simulink model "lab6"  (R2019b)
settings: Solver=FixedStepDiscrete  StartTime=0.0  StopTime=inf  RelTol=1e-3
values from neighbouring files (symbols this model uses):
  model_skory = createSkinModel2(RGB,BW)    [Lab6.m]
undefined symbols (not defined in the file or in its folder): gray, Rec, SDTV
libraries: visionconversions x1, visiontextngfix x1, dspvision x1
settings Model: Creator=fw2ty  LastModifiedBy=fw2ty

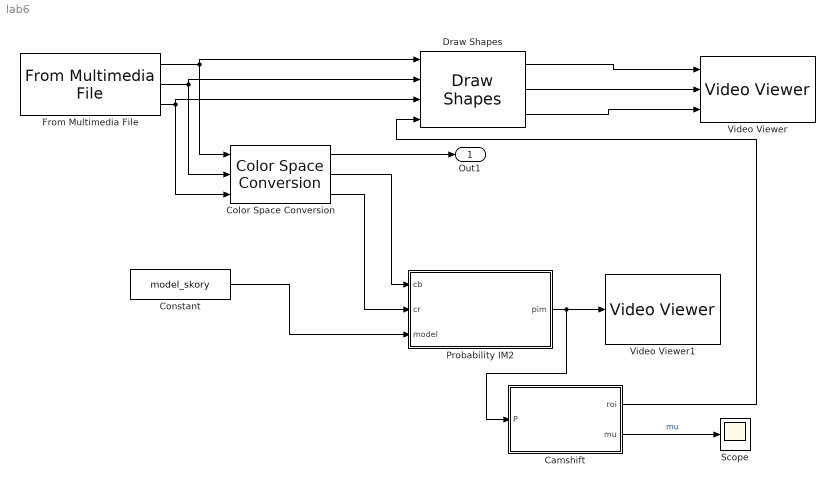
== system lab6 ==
  Camshift : MATLAB Function  TreatAsAtomicUnit=on
  Color Space Conversion : visionconversions/Color Space  Conversion  conversion=Obsolete  conversionActive=R'G'B' to Y'CbCr  wp_str=D65  rec=Rec. 601 (SDTV)  sys=1125/60/2:1  imagePorts=Separate color signals
  Constant : Constant  Value=model_skory
  Draw Shapes : visiontextngfix/Draw Shapes  shape=Rectangles  fill=off  lineWidth=1  fillClrSource=Specify via dialog  display=Black  intensity=200  color=[200 255 100]  opacity=0.6  viewport=Entire image  antialiasing=off  inType=Obsolete  imagePorts=Separate color signals  roundingMode=Floor  overflowMode=off  memoryMode=Specify word length  memoryWordLength=16  prodOutputMode=Binary point scaling  prodOutputWordLength=32  prodOutputFracLength=14  prodOutputSlope=2^-14  accumSlope=2^-14  memoryFracLength=15
      settings: SourceProductName=Computer Vision Toolbox
  From Multimedia File : dspvision/From Multimedia File  inputFilename=video.avi  readRange=[1 Inf]  loop=on  numPlays=inf  outputStreams=Video only  videoDataType=uint8  audioDataType=int16  inheritSampleTime=on  userDefinedSampleTime=1/30  noAudioOutput=off  isIntensityVideo=off  fourcc=RGB  colorVideoFormat=Separate color signals  outputEOF=off  dataOrg=Column-major  audioFrameSize=1024  computeAudioFrameSize=off  outSamplingMode=Sample based
      settings: SourceProductName=DSP System Toolbox  SourceProductBaseCode=DS
  Probability IM2 : MATLAB Function  TreatAsAtomicUnit=on
  Scope : Scope
  Video Viewer : VideoViewer  imagePorts=separate color signals  colormapValue=gray(256)  FigPos=[370 695 408 302]
  Video Viewer1 : VideoViewer  useColorMap=on  specRange=on  maxInputVal=1  FigPos=[845 857 587 499]
  Out1 : Outport
  wires:
  From Multimedia File/1 -> Draw Shapes/1, Color Space Conversion/1
  From Multimedia File/2 -> Color Space Conversion/2, Draw Shapes/2
  From Multimedia File/3 -> Color Space Conversion/3, Draw Shapes/3
  Color Space Conversion/2 -> Probability IM2/1(cb)
  Color Space Conversion/3 -> Probability IM2/2(cr)
  Constant/1 -> Probability IM2/3(model)
  Probability IM2/1(pim) -> Camshift/1(P), Video Viewer1/1
  Color Space Conversion/1 -> Out1/1
  Camshift/1(roi) -> Draw Shapes/4
  Draw Shapes/1 -> Video Viewer/1
  Draw Shapes/2 -> Video Viewer/2
  Draw Shapes/3 -> Video Viewer/3
  Camshift/2(mu) -> Scope/1  "mu"

== matlab function lab6/Probability IM2 ==
  data: cb input; cr input; model input; pim output
function pim = probabilityIM2(cb,cr,model)
    ind=sub2ind([256 256],cb(:),cr(:));
    outim=model(ind);
    pim=reshape(outim,size(cb(:,:,1)));

== matlab function lab6/Camshift ==
  data: P input; roi output; mu output
function [roi,mu]=Camshift(P)
%#codegen
% Uproszczony algorytm CAMSHIFT
%
% INPUT:
% > P       - obraz prawdopodobienstwa <0-1>
% OUTPUT:                                                                         
% > roi     - wspolrzedne ROI sledzonego obiektu [x,y,w,h]
% > mu      - wspolrzedne srodka ROI [x,y]
%
% DEPENDICIES:
% -
% COMMENTS:
% > TODO kontrola argumentow wejsciowych oraz optymalizacja kodu pod
%   wzgledem szybkosci
% CREATED: Jaromir Przybylo, 26.10.2015, R2015a
% LASTMODIFIED: 
%

% Inicjalizacja
S = -100;
Sp = 100;
[m,n]=size(P);
[mm,nn]=meshgrid(1:n,1:m);
P1=double(P);
BW=ones(m,n);
mm1=mm;nn1=nn;
roi  = uint32([1 1 m n]);
MU=uint32([m/2 n/2]);

% Camshift (bardzo uproszczony)
while abs(S-Sp)>1
    Sp=S;
    P1=P.*BW;
    mm1=mm.*BW;
    nn1=nn.*BW;
    
    m00=sum(sum(P1));
    m10=sum(sum(P1.*mm1));
    m01=sum(sum(P1.*nn1));
    
    MU=uint32([m10/m00 m01/m00]);
    S=2*sqrt(1*m00/1);
    
    min1=max([round(MU-S/2);1 1]);
    max1=min([round(MU+S/2);n m]);
    
    roi  = uint32([MU(1)-S/2 MU(2)-S/2 S S]);
    
    BW=zeros(m,n);
    BW(min1(2):max1(2),min1(1):max1(1))=1;    
end      

roi=roi;
mu=MU;
